simulink model "mrdamper"  (R2014a)
settings: Solver=ode45  SolverName=ode3  SolverMode=SingleTasking  StartTime=start_time  StopTime=stop_time  FixedStep=min_step  RelTol=1e-3
undefined symbols (not defined in the file): A, alpha_a, alpha_b, amp, beta, c, c0_a, c0_b, c1_a, c1_b, delta_t, g, gama, initial_disp, initial_velocity, k, k0, k1, m, n, noo, switchF, target_t
libraries: simulink x1, fuzblock x1
settings Model: CovMetricSettings=dwe  CovHtmlReporting=off  covSaveCumulativeToWorkspaceVar=off  CovSaveSingleToWorkspaceVar=off  CovExternalEMLEnable=on  CovSFcnEnable=on  Creator=mehrab  LastModifiedBy=mehrab
settings DataIOCC: LimitDataPoints=off  SaveFormat=StructureWithTime
settings DebuggingCC: MergeDetectMultiDrivingBlocksExec=error  SolverPrmCheckMsg=none  FrameProcessingCompatibilityMsg=error  SFUnexpectedBacktrackingDiag=error  SFNoUnconditionalDefaultTransitionDiag=error
settings HardwareCC: ProdBitPerPointer=64  ProdLargestAtomicFloat=Float  ProdIntDivRoundTo=Zero  ProdEndianess=LittleEndian  ProdHWDeviceType=Specified
settings ModelReferenceCC: PropagateSignalLabelsOutOfModel=on
settings GRTTargetCC: TargetLangStandard=C99 (ISO)

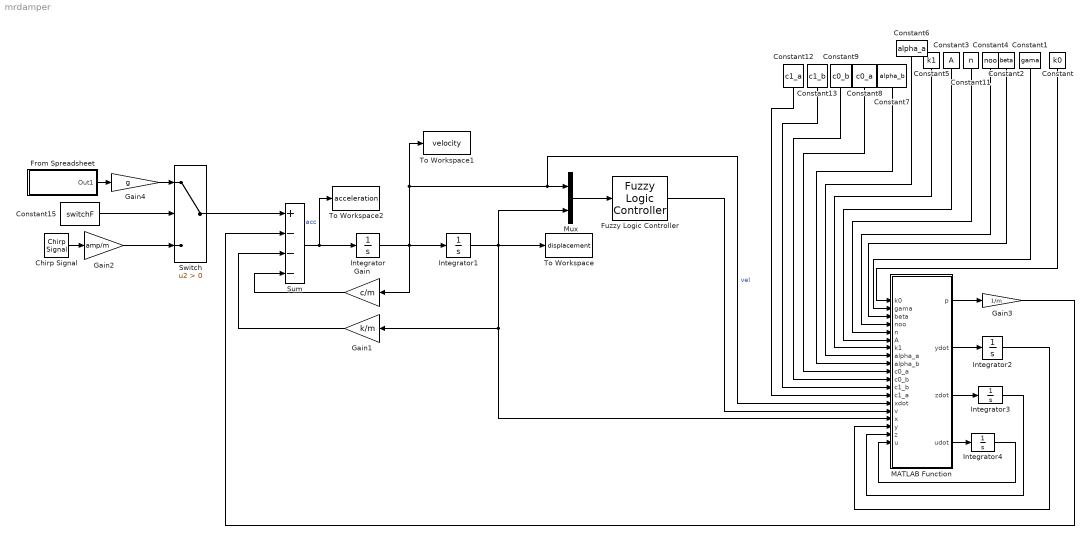
== system mrdamper ==
  Chirp Signal : simulink/Sources/Chirp Signal  f1=initial_freq  T=target_t  f2=freq_target
  Constant : Constant  Value=k0  VectorParams1D=off  OutDataTypeStr=double
  Constant1 : Constant  Value=gama  VectorParams1D=off  OutDataTypeStr=double
  Constant11 : Constant  Value=n  VectorParams1D=off  OutDataTypeStr=double
  Constant12 : Constant  Value=c1_a  VectorParams1D=off  OutDataTypeStr=double
  Constant13 : Constant  Value=c1_b  VectorParams1D=off  OutDataTypeStr=double
  Constant15 : Constant  Value=switchF
  Constant2 : Constant  Value=beta  VectorParams1D=off  OutDataTypeStr=double
  Constant3 : Constant  Value=A  VectorParams1D=off  OutDataTypeStr=double
  Constant4 : Constant  Value=noo  VectorParams1D=off  OutDataTypeStr=double
  Constant5 : Constant  Value=k1  VectorParams1D=off  OutDataTypeStr=double
  Constant6 : Constant  Value=alpha_a  VectorParams1D=off  OutDataTypeStr=double
  Constant7 : Constant  Value=alpha_b  VectorParams1D=off  OutDataTypeStr=double
  Constant8 : Constant  Value=c0_a  VectorParams1D=off  OutDataTypeStr=double
  Constant9 : Constant  Value=c0_b  VectorParams1D=off  OutDataTypeStr=double
  From Spreadsheet : Subsystem  Description=Replaced Block  mask(Replaced Block){}
      mask help: This block has been replaced with an empty subsystem because it used functionality that is unavailable in Simulink R2014a.
      mask Display: fprintf('Replaced: %s\n','FromSpreadsheet')
  Fuzzy Logic Controller : fuzblock/Fuzzy Logic  Controller  FIS='mrfuzzy'
  Gain : Gain  Gain=c/m
  Gain1 : Gain  Gain=k/m
  Gain2 : Gain  Gain=amp/m
  Gain3 : Gain  Gain=1/m
  Gain4 : Gain  Gain=g
  Integrator : Integrator  InitialCondition=initial_velocity
  Integrator1 : Integrator  InitialCondition=initial_disp
  Integrator2 : Integrator
  Integrator3 : Integrator
  Integrator4 : Integrator
  MATLAB Function : MATLAB Function  TreatAsAtomicUnit=on
      settings: PermitHierarchicalResolution=ParametersOnly
  Mux : Mux  Inputs=2
  Sum : Sum  Inputs=+---
  Switch : Switch  Criteria=u2 > Threshold
  To Workspace : ToWorkspace  VariableName=displacement  SampleTime=delta_t
  To Workspace1 : ToWorkspace  VariableName=velocity  SampleTime=delta_t
  To Workspace2 : ToWorkspace  VariableName=acceleration  SampleTime=delta_t
  wires:
  Chirp Signal/1 -> Gain2/1
  Sum/1 -> To Workspace2/1, Integrator/1  "acc"
  Integrator/1 -> To Workspace1/1, MATLAB Function/14(xdot), Mux/1, Gain/1, Integrator1/1  "vel"
  Gain/1 -> Sum/4
  Gain1/1 -> Sum/3
  Mux/1 -> Fuzzy Logic Controller/1
  Fuzzy Logic Controller/1 -> MATLAB Function/15(v)
  MATLAB Function/3(zdot) -> Integrator3/1
  MATLAB Function/2(ydot) -> Integrator2/1
  Integrator2/1 -> MATLAB Function/17(y)
  Integrator3/1 -> MATLAB Function/18(z)
  MATLAB Function/1(p) -> Gain3/1
  Gain3/1 -> Sum/2
  Integrator1/1 -> To Workspace/1, Gain1/1, MATLAB Function/16(x), Mux/2
  MATLAB Function/4(udot) -> Integrator4/1
  Integrator4/1 -> MATLAB Function/19(u)
  Constant9/1 -> MATLAB Function/11(c0_b)
  Constant8/1 -> MATLAB Function/10(c0_a)
  Constant7/1 -> MATLAB Function/9(alpha_b)
  Constant5/1 -> MATLAB Function/7(k1)
  Constant3/1 -> MATLAB Function/6(A)
  Constant11/1 -> MATLAB Function/5(n)
  Constant4/1 -> MATLAB Function/4(noo)
  Constant2/1 -> MATLAB Function/3(beta)
  Constant1/1 -> MATLAB Function/2(gama)
  Constant/1 -> MATLAB Function/1(k0)
  Constant6/1 -> MATLAB Function/8(alpha_a)
  Constant13/1 -> MATLAB Function/12(c1_b)
  Constant12/1 -> MATLAB Function/13(c1_a)
  Switch/1 -> Sum/1
  Gain2/1 -> Switch/3
  Constant15/1 -> Switch/2
  Gain4/1 -> Switch/1
  From Spreadsheet/1(Out1) -> Gain4/1

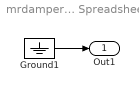
== system mrdamper/From Spreadsheet ==
  Ground1 : Ground
  Out1 : Outport
  wires:
  Ground1/1 -> Out1/1

== matlab function mrdamper/MATLAB Function ==
  data: k0 input; gama input; beta input; noo input; n input; A input; k1 input; alpha_a input; alpha_b input; c0_a input; c0_b input; c1_b input; c1_a input; p output; xdot input; v input; x input; ydot output; y input; z input; zdot output; u input; udot output
function [p,ydot,zdot,udot] = fcn(k0,gama,beta,noo,n, A,k1,alpha_a,alpha_b,c0_a,c0_b,c1_b,c1_a,xdot,v,x,y,z,u)

udot=-noo*(u-v);
alpha=alpha_a+alpha_b*u;
c0=c0_a+c0_b*u;
c1=c1_a+c1_b*u;



ydot=(1/(c0+c1))*(alpha*z+c0*xdot+k0*(x-y));
zdot=-gama*abs(xdot-ydot)*z*abs(z)^(n-1)-beta*(xdot-ydot)*(abs(z))^n+A*(xdot-ydot);
P=c1*ydot+k1*(x);
p=alpha*z+c0*(xdot-ydot)+k0*(x-y)+k1*(x-0.18);
end
